simulink model "temp_gen_pch"  (R2025b)
settings: Solver=ode4  StartTime=0.0  StopTime=45  FixedStep=0.01  RelTol=1e-3  EnableMultiTasking=on
settings Model: Creator=oravec  LastModifiedBy=juroo
settings SolverCC: AlgebraicLoopSolver=TrustRegion
settings DataIOCC: SaveFormat=Array  SignalLoggingSaveFormat=ModelDataLogs  ReturnWorkspaceOutputs=off  SignalLoggingName=sigsOut
settings OptimizationCC: LifeSpan=inf
settings DebuggingCC: SaveWithParameterizedLinksMsg=none  UnderspecifiedInitializationDetection=Classic  MergeDetectMultiDrivingBlocksExec=none  SignalResolutionControl=TryResolveAllWithWarning  MultiTaskDSMMsg=warning  MultiTaskCondExecSysMsg=none  FcnCallInpInsideContextMsg=warning  UnconnectedInputMsg=warning  UnconnectedOutputMsg=warning  UnconnectedLineMsg=warning  SFUnexpectedBacktrackingDiag=warning  SFNoUnconditionalDefaultTransitionDiag=warning  SFExecutionAtInitializationDiag=none  ArithmeticOperatorsInVariantConditions=warning
settings HardwareCC: ProdBitPerPointer=32.0  ProdBitPerSizeT=32.0  ProdBitPerPtrDiffT=32.0  ProdLargestAtomicFloat=None  ProdIntDivRoundTo=Undefined  ProdEndianess=Unspecified  ProdWordSize=32.0  ProdHWDeviceType=32-bit Generic  TargetHWDeviceType=32-bit Generic  TargetUnknown=on  ProdEqTarget=off
settings ModelReferenceCC: EnableRefExpFcnMdlSchedulingChecks=on  PropagateSignalLabelsOutOfModel=off
settings RTWCC: GPUComputeCapability=3.5  DLArmComputeVersion=19.05
settings CodeAppCC: StateflowObjectComments=on
settings GRTTargetCC: TargetFcnLib=ansi_tfl_tmw.mat  TargetLangStandard=C89/C90 (ANSI)  CombineOutputUpdateFcns=off  GRTInterface=on
settings ConfigComp: CovMetricSettings=dw  CovSaveCumulativeToWorkspaceVar=on  CovSaveSingleToWorkspaceVar=on

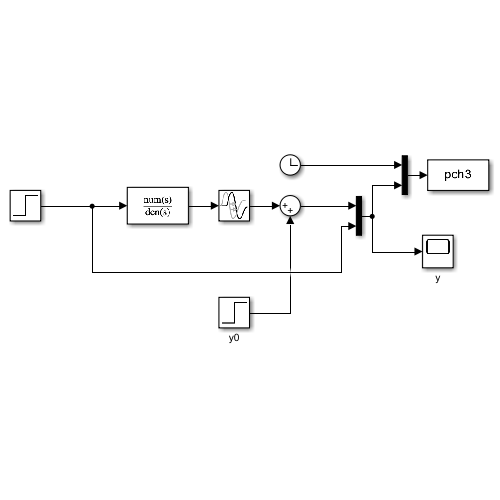
[thumbnail: Simulink's stored preview of the top-level diagram]
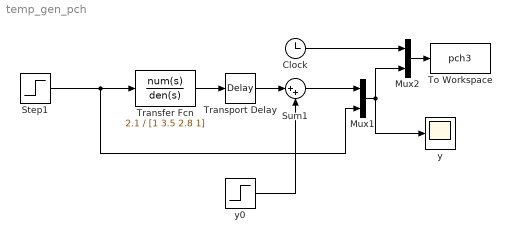
== system temp_gen_pch ==
  Clock : Clock
  Mux1 : Mux  Inputs=2
  Mux2 : Mux  Inputs=2
  Step1 : Step  Time=0  Before=-1  After=2  SampleTime=0
  Sum1 : Sum  Inputs=|++
  To Workspace : ToWorkspace  VariableName=pch3  SampleTime=-1
  Transfer Fcn : TransferFcn  Numerator=2.1  Denominator=[1 3.5 2.8 1]
  Transport Delay : TransportDelay  DelayTime=0.3
  y : Scope
      settings: DataLoggingVariableName=ScopeData2
  y0 : Step  Time=0  After=3  SampleTime=0
  wires:
  Transfer Fcn/1 -> Transport Delay/1
  Mux1/1 -> y/1, Mux2/2
  Transport Delay/1 -> Sum1/1
  y0/1 -> Sum1/2
  Mux2/1 -> To Workspace/1
  Sum1/1 -> Mux1/1
  Clock/1 -> Mux2/1
  Step1/1 -> Transfer Fcn/1, Mux1/2
